simulink model "RL_Generated"  (R2024b)
settings: Solver=FixedStepAuto  StartTime=0  StopTime=5  FixedStep=Ts  RelTol=1e-3
undefined symbols (not defined in the file or in its folder): ApparatusPara, PowerFlow, Ts, Wbase, Zbase
libraries: SimplusGT x4, spsGroundLib x2, spsThreePhaseSeriesRLCBranchLib x1, sps_lib x1
settings Model: Creator=gzhan  LastModifiedBy=gzhan

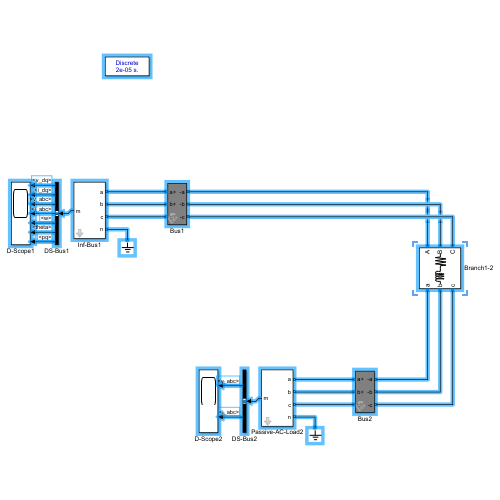
[thumbnail: Simulink's stored preview of the top-level diagram]
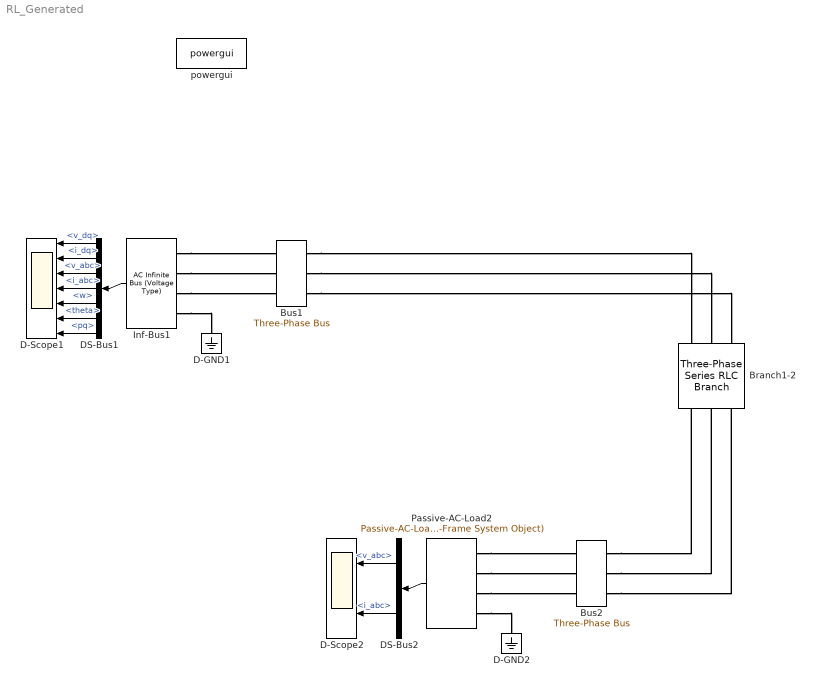
== system RL_Generated ==
  Branch1-2 : spsThreePhaseSeriesRLCBranchLib/Three-Phase Series RLC Branch  LConnTagsString=A|B|C  RConnTagsString=A|B|C  BranchType=RL  Resistance=(0.02)*Zbase  Inductance=(0.1)*Zbase/Wbase  Capacitance=1e-6  Measurements=None
  Bus1 : SimplusGT/Three-Phase Bus  Vbase=1  Sbase=1
  Bus2 : SimplusGT/Three-Phase Bus  Vbase=1  Sbase=1
  D-GND1 : spsGroundLib/Ground  LConnTagsString=a
  D-GND2 : spsGroundLib/Ground  LConnTagsString=a
  D-Scope1 : Scope  NumInputPorts=7
  D-Scope2 : Scope  NumInputPorts=2
  DS-Bus1 : BusSelector  OutputSignals=v_dq,i_dq,v_abc,i_abc,w,theta,pq
  DS-Bus2 : BusSelector  OutputSignals=v_abc,i_abc
  Inf-Bus1 : SimplusGT/AC Infinite Bus (Voltage Type)  Ts=Ts  Sbase=Sbase  Vbase=Vbase  Wbase=Wbase  vd=PowerFlow{1}(3)  vq=0  theta0=PowerFlow{1}(4)  w=Wbase  R=1e-30
  Passive-AC-Load2 : SimplusGT/Passive-AC-Load (dq-Frame System Object)  Sbase=Sbase  Vbase=Vbase  Wbase=Wbase  ApparatusPara=ApparatusPara{2}  Ts=Ts
  powergui : sps_lib/powergui  Priority=1  SimulationMode=Discrete  SampleTime=Ts  frequency=60  Iterations=50  frequencyindice=0  Pbase=100e6  ErrMax=1e-4  UnitsV=kV  UnitsW=MW  buscounter=0  FunctionMessages=off  echomessages=off  EnableUseOfTLC=off  CurrentSourceSwitches=off  DisableSnubberDevices=off  DisableRonSwitches=off  DisableVfSwitches=off  DisplayEquations=off  AutomaticDiscreteSolvers=off  SolverType=Tustin/Backward Euler (TBE)  Interpol=off  ExternalGateDelay=off  methode=off  Ts=100  x0status=blocks  SPID=on  SwTol=0  HookPort=off  NonlinearTolerance=1e-4  nMaxIteration=100  ContinueOnMaxIteration=off  RestoreLinks=warning  ResistiveCurrentMeasurement=off  Frange=[0:2:500]  Ylog=off  Xlog=on  ShowGrid=off  save=off  variable=ZData  structure=0  ZoomFFT=off  StartTime=0.0  cycles=1  DisplayStyle=1  fundamental=60  FreqAxis=off  MaxFrequency=1000  frequencyindicesteady=1  RmsSteady=1  display=off
  wires:
  Inf-Bus1/1 -> DS-Bus1/1
  DS-Bus1/1 -> D-Scope1/1  "<v_dq>"
  DS-Bus1/2 -> D-Scope1/2  "<i_dq>"
  DS-Bus1/3 -> D-Scope1/3  "<v_abc>"
  DS-Bus1/4 -> D-Scope1/4  "<i_abc>"
  DS-Bus1/5 -> D-Scope1/5  "<w>"
  DS-Bus1/6 -> D-Scope1/6  "<theta>"
  DS-Bus1/7 -> D-Scope1/7  "<pq>"
  Passive-AC-Load2/1 -> DS-Bus2/1
  DS-Bus2/1 -> D-Scope2/1  "<v_abc>"
  DS-Bus2/2 -> D-Scope2/2  "<i_abc>"
  connections:
  Inf-Bus1/LConn4 -- D-GND1/LConn1
  Passive-AC-Load2/LConn4 -- D-GND2/LConn1
  Bus2/RConn1 -- Branch1-2/RConn1
  Bus2/RConn2 -- Branch1-2/RConn2
  Bus2/RConn3 -- Branch1-2/RConn3
  Bus1/RConn1 -- Branch1-2/LConn1
  Bus1/RConn2 -- Branch1-2/LConn2
  Bus1/RConn3 -- Branch1-2/LConn3
  Inf-Bus1/LConn1 -- Bus1/LConn1
  Inf-Bus1/LConn2 -- Bus1/LConn2
  Inf-Bus1/LConn3 -- Bus1/LConn3
  Passive-AC-Load2/LConn1 -- Bus2/LConn1
  Passive-AC-Load2/LConn2 -- Bus2/LConn2
  Passive-AC-Load2/LConn3 -- Bus2/LConn3
